simulink model "Monitorizacion"  (R2022a)
settings: Solver=FixedStepAuto  StartTime=0.0  StopTime=inf  FixedStep=0.01  RelTol=1e-1
values from neighbouring files (symbols this model uses):
  AD = 0    [plotEnsayosPC.m]
  b = 0.8    [plotEnsayosPC.m]
  K = 7.27    [plotEnsayosPC.m]
  N = 5    [plotEnsayosPC.m]
  Td = 0    [plotEnsayosPC.m]
  Ti = 0.065    [plotEnsayosPC.m]
undefined symbols (not defined in the file or in its folder): angular, linear
libraries: ros2lib x7, dspsigops x1
settings Model: Creator=Francisco  LastModifiedBy=Francisco
settings OptimizationCC: EnhancedBackFolding=on  PassReuseOutputArgsAs=Individual arguments  ZeroExternalMemoryAtStartup=off  ZeroInternalMemoryAtStartup=off  MaxStackSize=64  OptimizeBlockOrder=speed  DifferentSizesBufferReuse=on  OptimizationCustomize=off  EfficientTunableParamExpr=on
settings DebuggingCC: ParameterTunabilityLossMsg=error
settings SFSimCC: MATLABDynamicMemAlloc=off
settings RTWCC: SystemTargetFile=ert.tlc  HardwareBoard=Robot Operating System 2 (ROS 2)  TLCOptions="-aInlineSetEventsForThisBaseRateFcn=TLC_FALSE -aSuppressMultiTaskScheduler=TLC_FALSE  -aRateBasedStepFcn=0"  TemplateMakefile=ert_default_tmf  Toolchain=Colcon Tools  TargetLang=C++
settings CodeAppCC: ForceParamTrailComments=on  IgnoreCustomStorageClasses=off  OperatorAnnotations=on  SimulinkDataObjDesc=on  SFDataObjDesc=on  InsertBlockDesc=on
settings ERTTargetCC: CodeInterfacePackaging=C++ class  RootIOFormat=Structure reference

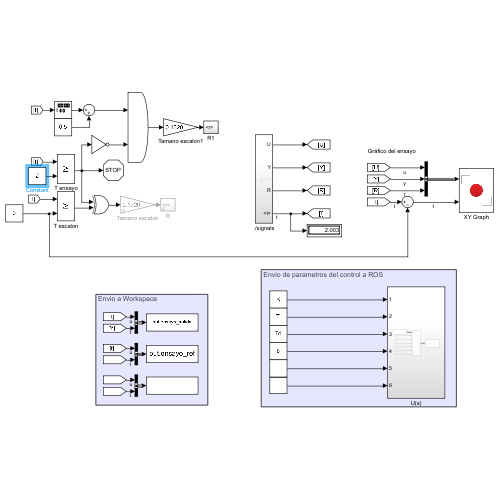
[thumbnail: Simulink's stored preview of the top-level diagram]
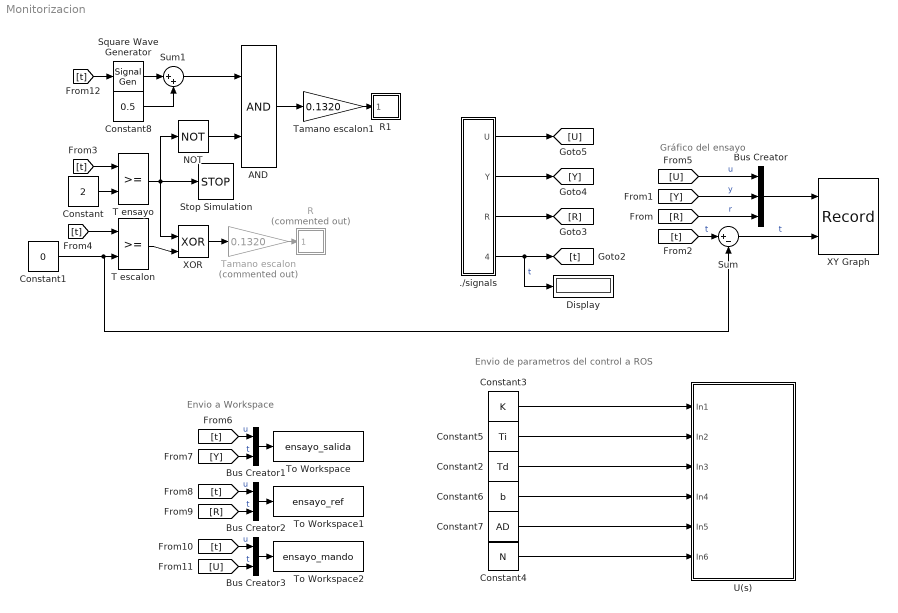
== system Monitorizacion ==
  note: Gráfico del ensayo
  note: Envio de parametros del control a ROS
  note: Envio a Workspace
  ./signals : Subsystem
  AND : Logic  IconShape=distinctive  AllPortsSameDT=off  OutDataTypeStr=boolean
  Bus Creator : BusCreator  Inputs=3
  Bus Creator1 : BusCreator  Inputs=2
  Bus Creator2 : BusCreator  Inputs=2
  Bus Creator3 : BusCreator  Inputs=2
  Constant : Constant  Value=2
  Constant1 : Constant  Value=0
  Constant2 : Constant  Value=Td
  Constant3 : Constant  Value=K
  Constant4 : Constant  Value=N
  Constant5 : Constant  Value=Ti
  Constant6 : Constant  Value=b
  Constant7 : Constant  Value=AD
  Constant8 : Constant  Value=0.5
  Display : Display
  NOT : Logic  Operator=NOT  IconShape=distinctive  AllPortsSameDT=off  OutDataTypeStr=boolean
  R : Subsystem  Commented=on
  R1 : Subsystem
  Square Wave Generator : SignalGenerator  WaveForm=square  TimeSource=Use external signal  Amplitude=0.5  Frequency=1/2
  Stop Simulation : Stop
  Sum : Sum  Inputs=|+-
  Sum1 : Sum  Inputs=|++
  T ensayo : RelationalOperator  OutDataTypeStr=boolean  RndMeth=Simplest  InputSameDT=off
  T escalon : RelationalOperator  OutDataTypeStr=boolean  RndMeth=Simplest  InputSameDT=off
  Tamano escalon : Gain  Commented=on  Gain=0.1320  OutDataTypeStr=double
  Tamano escalon1 : Gain  Gain=0.1320  OutDataTypeStr=double
  To Workspace : ToWorkspace  VariableName=ensayo_salida  SampleTime=-1
  To Workspace1 : ToWorkspace  VariableName=ensayo_ref  SampleTime=-1
  To Workspace2 : ToWorkspace  VariableName=ensayo_mando  SampleTime=-1
  U(s) : Subsystem
  XOR : Logic  Operator=XOR  IconShape=distinctive  AllPortsSameDT=off  OutDataTypeStr=boolean
  XY Graph : Record  FileSettingsInternal="{\"entries\":[{\"content\":{\"excelSettings\":{\"content\":{},\"type\":\"Streamout.ExcelSettings\"}},\"type\":\"Streamout.FileSettingStorage\",\"uuid\":\"cd18d70d-eef8-43d3-8d9d-1d93410516e5\"}],\"packageUris\":[\"http://schema.mathworks.com/mf0/streamout_blocks/R2020a\"],\"version\":\"1.0\"}"  Layout=[2 1]  SignalsInternal="{\"entries\":[{\"content\":{\"signals\":[{\"content\":{\"blockPath\":[\"Monitorizacion/XY Graph\"],\"channel\":[],\"dimensions\":[1],\"domain\":\"Monitorizacion/XY Graph\",\"hasChildren\":true,\"lineColor\":\"#4dbeee\",\"plots\":[],\"port\":1,\"sid\":[\"\"],\"signalID\":7057,\"signalName\":\"Bus\\nCreator\"},\"type\":\"RecordBlkView.Signal\",\"uuid\":\"fd950e00-f479-4cde-be91-977f4fdee8a2\"},{\"content\":{\"blockPath\":[\"Monitorizacion/XY Graph\"],\"channel\":[],\"dimensions\":[1],\"domain\":\"Monitorizacion/XY Graph\",\"leafPath\":\"Bus\\nCreator.u\",\"lineColor\":\"#ff13a6\",\"parentID\":7057,\"plots\":[2],\"port\":1,\"sid\":[\"\"],\"signalID\":7063,\"signalName\":\"Bus\\nCreator.u\"},\"type\":\"RecordBlkView.Signal\",\"uuid\":\"f3818dbe-a55d-4531-a50d-b813396fe280\"},{\"content\":{\"blockPath\":[\"Monitorizacion/XY Graph\"],\"channel\":[],\"dimensions\":[1],\"domain\":\"Monitorizacion/XY Graph\",\"leafPath\":\"Bus\\nCreator.y\",\"lineColor\":\"#b746ff\",\"parentID\":7057,\"plots\":[1],\"port\":1,\"sid\":[\"\"],\"signalID\":7067,\"signalName\":\"Bus\\nCreator.y\"},\"type\":\"RecordBlkView.Signal\",\"uuid\":\"d2dda603-44a7-4e1b-afdf-04a08ad27c0b\"},{\"content\":{\"blockPath\":[\"Monitorizacion/XY Graph\"],\"channel\":[],\"dimensions\":[1],\"domain\":\"Monitorizacion/XY Graph\",\"leafPath\":\"Bus\\nCreator.r\",\"lineColor\":\"#22b573\",\"parentID\":7057,\"plots\":[1],\"port\":1,\"sid\":[\"\"],\"signalID\":7071,\"signalName\":\"Bus\\nCreator.r\"},\"type\":\"RecordBlkView.Signal\",\"uuid\":\"0c59df63-b69a-4317-a54f-8d2f4f2e6e05\"},{\"content\":{\"blockPath\":[\"Monitorizacion/XY Graph\"],\"channel\":[],\"dimensions\":[1],\"domain\":\"Monitorizacion/XY Graph\",\"lineColor\":\"#139fff\",\"plots\":[2,1],\"port\":2,\"sid\":[\"\"],\"signalID\":7073,\"signalName\":\"t\"},\"type\":\"RecordBlkView.Signal\",\"uuid\":\"04769aad-d8d1-45e3-899e-6b90242f4b2a\"}]},\"type\":\"RecordBlkView.InputSignals\",\"uuid\":\"ca370a18-30cd-4c71-8227-67b3cc56881f\"}],\"packageUris\":[\"http://schema.mathworks.com/mf0/streamout_blocks/R2020a\"],\"version\":\"1.0\"}"  VisualizationBindings="{\"xyplotplugin\":{\"info\":[{\"series\":[{\"bindingParametersList\":[{\"parameter\":\"X-Axis\",\"signalID\":7073,\"signalName\":\"t\"},{\"parameter\":\"Y-Axis\",\"signalID\":7067,\"signalName\":\"Bus\\nCreator.y\"}],\"seriesID\":29406},{\"bindingParametersList\":[{\"parameter\":\"X-Axis\",\"signalID\":7073,\"signalName\":\"t\"},{\"parameter\":\"Y-Axis\",\"signalID\":7071,\"signalName\":\"Bus\\nCreator.r\"}],\"seriesID\":15878}],\"subplotID\":1},{\"series\":[{\"bindingParametersList\":[{\"parameter\":\"X-Axis\",\"signalID\":7073,\"signalName\":\"t\"},{\"parameter\":\"Y-Axis\",\"signalID\":7063,\"signalName\":\"Bus\\nCreator.u\"}],\"seriesID\":22894}],\"subplotID\":2}]}}"  CompatibilityTag=XY
  wires:
  [t] -> T ensayo/1
  Constant/1 -> T ensayo/2
  [t] -> T escalon/1
  XOR/1 -> Tamano escalon/1
  T escalon/1 -> XOR/2
  Tamano escalon/1 -> R/1(<r>)
  ./signals/1(U) -> [U]
  ./signals/2(Y) -> [Y]
  ./signals/3(R) -> [R]
  Bus Creator/1 -> XY Graph/1
  [R] -> Bus Creator/3  "r"
  [Y] -> Bus Creator/2  "y"
  [U] -> Bus Creator/1  "u"
  ./signals/4(<t>) -> Display/1, [t]  "t"
  Sum/1 -> XY Graph/2  "t"
  Constant1/1 -> Sum/2, T escalon/2
  [t] -> Sum/1  "t"
  T ensayo/1 -> XOR/1, NOT/1, Stop Simulation/1
  Bus Creator3/1 -> To Workspace2/1
  [U] -> Bus Creator3/2  "t"
  [Y] -> Bus Creator1/2  "t"
  [t] -> Bus Creator2/1  "u"
  [t] -> Bus Creator1/1  "u"
  Bus Creator1/1 -> To Workspace/1
  [R] -> Bus Creator2/2  "t"
  [t] -> Bus Creator3/1  "u"
  Bus Creator2/1 -> To Workspace1/1
  Constant7/1 -> U(s)/5(In5)
  Constant5/1 -> U(s)/2(In2)
  Constant3/1 -> U(s)/1(In1)
  Constant6/1 -> U(s)/4(In4)
  Constant4/1 -> U(s)/6(In6)
  Constant2/1 -> U(s)/3(In3)
  Constant8/1 -> Sum1/2
  [t] -> Square Wave Generator/1
  Square Wave Generator/1 -> Sum1/1
  NOT/1 -> AND/2
  Sum1/1 -> AND/1
  Tamano escalon1/1 -> R1/1(<r>)
  AND/1 -> Tamano escalon1/1

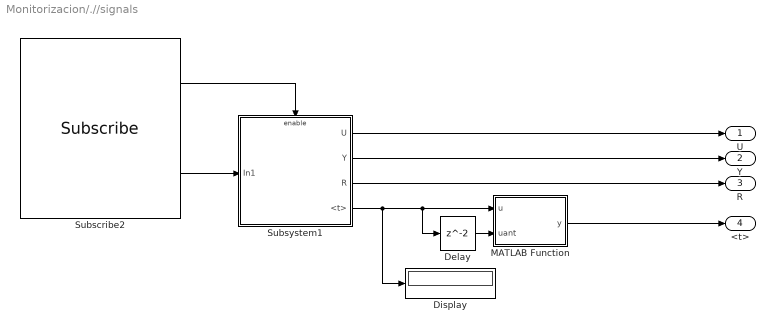
== system Monitorizacion/.//signals ==
  Delay : Delay
  Display : Display
  MATLAB Function : MATLAB Function  TreatAsAtomicUnit=on
  Subscribe2 : ros2lib/Subscribe  topicSource=Specify your own  topic=/signals  messageType=geometry_msgs/TwistStamped  sampleTime=-1  QOSHistory=Keep last  QOSDepth=10  QOSReliability=Best effort  QOSDurability=Volatile
      settings: SourceProductBaseCode=RR
  Subsystem1 : Subsystem
  U : Outport
  Y : Outport  Port=2
  R : Outport  Port=3
  <t> : Outport  Port=4
  wires:
  Subscribe2/1 -> Subsystem1/Enable
  Subscribe2/2 -> Subsystem1/1(In1)
  Subsystem1/4(<t>) -> Display/1, Delay/1, MATLAB Function/1(u)
  Subsystem1/3(R) -> R/1
  Subsystem1/2(Y) -> Y/1
  Subsystem1/1(U) -> U/1
  Delay/1 -> MATLAB Function/2(uant)
  MATLAB Function/1(y) -> <t>/1

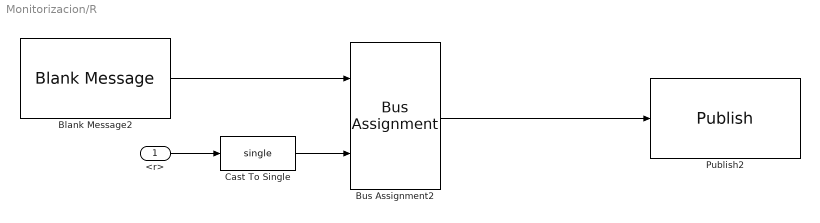
== system Monitorizacion/R ==
  <r> : Inport
  Blank Message2 : ros2lib/Blank Message  messageClass=Message  entityType=std_msgs/Float32  messageType=std_msgs/Float32  SampleTime=inf
      settings: SourceProductBaseCode=RR
  Bus Assignment2 : BusAssignment  AssignedSignals=data
  Cast To Single : DataTypeConversion  OutDataTypeStr=single  SaturateOnIntegerOverflow=off  RndMeth=Floor
  Publish2 : ros2lib/Publish  topicSource=Specify your own  topic=/ref  messageType=std_msgs/Float32  QOSHistory=Keep last  QOSDepth=1  QOSReliability=Reliable  QOSDurability=Volatile
      settings: SourceProductBaseCode=RR
  wires:
  Bus Assignment2/1 -> Publish2/1
  Blank Message2/1 -> Bus Assignment2/1
  <r>/1 -> Cast To Single/1
  Cast To Single/1 -> Bus Assignment2/2

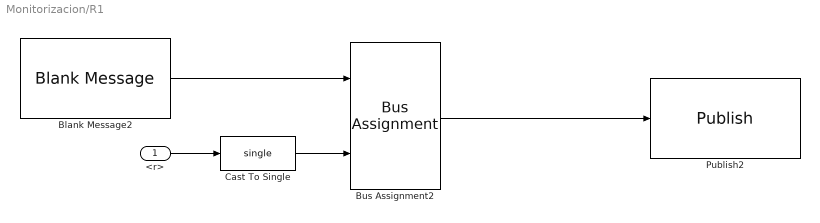
== system Monitorizacion/R1 ==
  <r> : Inport
  Blank Message2 : ros2lib/Blank Message  messageClass=Message  entityType=std_msgs/Float32  messageType=std_msgs/Float32  SampleTime=inf
      settings: SourceProductBaseCode=RR
  Bus Assignment2 : BusAssignment  AssignedSignals=data
  Cast To Single : DataTypeConversion  OutDataTypeStr=single  SaturateOnIntegerOverflow=off  RndMeth=Floor
  Publish2 : ros2lib/Publish  topicSource=Specify your own  topic=/ref  messageType=std_msgs/Float32  QOSHistory=Keep last  QOSDepth=1  QOSReliability=Reliable  QOSDurability=Volatile
      settings: SourceProductBaseCode=RR
  wires:
  Bus Assignment2/1 -> Publish2/1
  Blank Message2/1 -> Bus Assignment2/1
  <r>/1 -> Cast To Single/1
  Cast To Single/1 -> Bus Assignment2/2

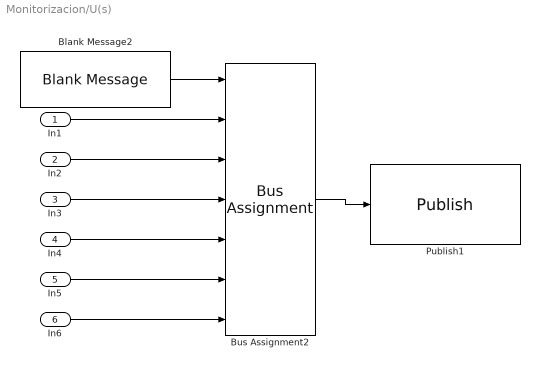
== system Monitorizacion/U(s) ==
  In1 : Inport
  In2 : Inport  Port=2
  In3 : Inport  Port=3
  In4 : Inport  Port=4
  In5 : Inport  Port=5
  In6 : Inport  Port=6
  Blank Message2 : ros2lib/Blank Message  messageClass=Message  entityType=geometry_msgs/Twist  messageType=geometry_msgs/Twist  SampleTime=inf
      settings: SourceProductBaseCode=RR
  Bus Assignment2 : BusAssignment  AssignedSignals=linear.x,linear.y,linear.z,angular.x,angular.y,angular.z
  Publish1 : ros2lib/Publish  topicSource=Select from ROS network  topic=/control  messageType=geometry_msgs/Twist  QOSHistory=Keep last  QOSDepth=1  QOSReliability=Reliable  QOSDurability=Volatile
      settings: SourceProductBaseCode=RR
  wires:
  Bus Assignment2/1 -> Publish1/1
  In1/1 -> Bus Assignment2/2
  In6/1 -> Bus Assignment2/7
  In2/1 -> Bus Assignment2/3
  Blank Message2/1 -> Bus Assignment2/1
  In4/1 -> Bus Assignment2/5
  In3/1 -> Bus Assignment2/4
  In5/1 -> Bus Assignment2/6

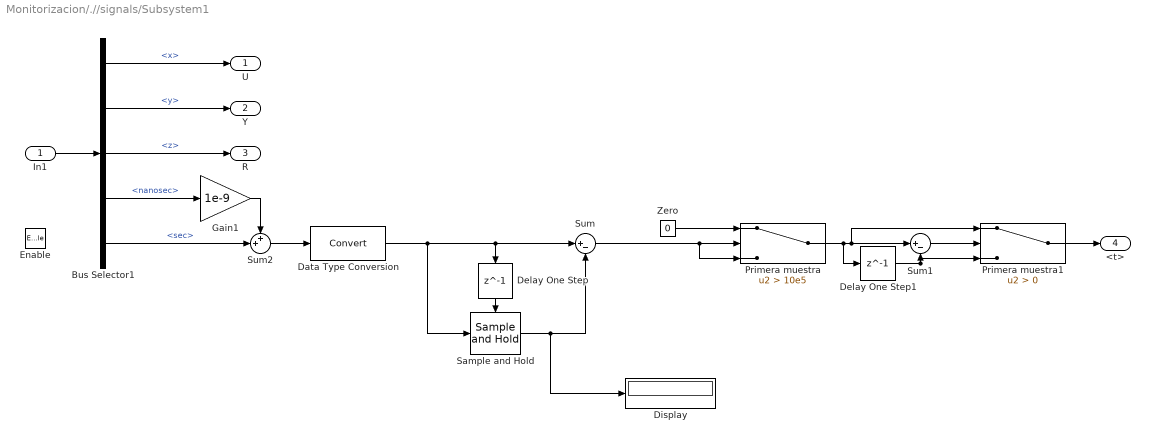
== system Monitorizacion/.//signals/Subsystem1 ==
  In1 : Inport
  Enable : EnablePort
  Bus Selector1 : BusSelector  OutputSignals=twist.linear.x,twist.linear.y,twist.linear.z,header.stamp.nanosec,header.stamp.sec
  Data Type Conversion : DataTypeConversion  SaturateOnIntegerOverflow=off  RndMeth=Floor
  Delay One Step : Delay  DelayLength=1
  Delay One Step1 : Delay  DelayLength=1
  Display : Display
  Gain1 : Gain  Gain=1e-9  OutDataTypeStr=double
  Primera muestra : Switch  Criteria=u2 > Threshold  Threshold=10e5  SaturateOnIntegerOverflow=off  InputSameDT=off
  Primera muestra1 : Switch  Criteria=u2 > Threshold  SaturateOnIntegerOverflow=off  InputSameDT=off
  Sample and Hold : dspsigops/Sample and Hold  trig=Rising edge  initCond=0  latchinput=off
  Sum : Sum  Inputs=|+-
  Sum1 : Sum  Inputs=|+-
  Sum2 : Sum  Inputs=++|
  Zero : Constant  Value=0  OutDataTypeStr=Inherit: Inherit via back propagation
  U : Outport
  Y : Outport  Port=2
  R : Outport  Port=3
  <t> : Outport  Port=4
  wires:
  In1/1 -> Bus Selector1/1
  Sum2/1 -> Data Type Conversion/1
  Gain1/1 -> Sum2/1
  Bus Selector1/5 -> Sum2/2  "<sec>"
  Bus Selector1/4 -> Gain1/1  "<nanosec>"
  Data Type Conversion/1 -> Sample and Hold/1, Sum/1, Delay One Step/1
  Bus Selector1/3 -> R/1  "<z>"
  Bus Selector1/2 -> Y/1  "<y>"
  Bus Selector1/1 -> U/1  "<x>"
  Delay One Step/1 -> Sample and Hold/Trigger
  Sample and Hold/1 -> Display/1, Sum/2
  Zero/1 -> Primera muestra/1
  Sum/1 -> Primera muestra/3, Primera muestra/2
  Primera muestra1/1 -> <t>/1
  Delay One Step1/1 -> Primera muestra1/3, Sum1/2
  Primera muestra/1 -> Delay One Step1/1, Primera muestra1/1, Sum1/1
  Sum1/1 -> Primera muestra1/2

== matlab function Monitorizacion/.//signals/MATLAB Function ==
  data: u input; y output; uant input
function y = fcn(u, uant)
    if(u>=uant)
        y=u;
    else
        y =uant;
    end
end
